simulink model "AnimationSpacecraftBodyVFC"  (R2020b)
settings: Solver=FixedStepDiscrete  StartTime=0.0  StopTime=inf  FixedStep=.1  RelTol=1e-3  EnableMultiTasking=on
InitFcn:
  | addpath('.')
libraries: simulink x6
settings Model: Creator=beard  LastModifiedBy=abdul
settings DataIOCC: LimitDataPoints=on  SaveFormat=Array  SignalLoggingSaveFormat=ModelDataLogs  ReturnWorkspaceOutputs=off
settings OptimizationCC: ExpressionDepthLimit=2147483647  InitFltsAndDblsToZero=on  LifeSpan=inf
settings DebuggingCC: UnderspecifiedInitializationDetection=Classic  MergeDetectMultiDrivingBlocksExec=none  SolverPrmCheckMsg=warning  FcnCallInpInsideContextMsg=warning  AllowSymbolicDim=off  StateNameClashWarn=warning  SFUnexpectedBacktrackingDiag=warning  SFNoUnconditionalDefaultTransitionDiag=warning  SFExecutionAtInitializationDiag=none  ArithmeticOperatorsInVariantConditions=warning
settings HardwareCC: ProdBitPerPointer=32  ProdBitPerSizeT=32  ProdBitPerPtrDiffT=32  ProdLargestAtomicFloat=None  ProdIntDivRoundTo=Undefined  ProdEndianess=Unspecified  ProdWordSize=32  ProdHWDeviceType=32-bit Generic
settings ModelReferenceCC: PropagateSignalLabelsOutOfModel=off
settings SFSimCC: SimUseLocalCustomCode=off  CustomCodeUndefinedFunction=UseInterfaceOnly
settings RTWCC: RTWUseLocalCustomCode=off
settings CodeAppCC: StateflowObjectComments=on
settings GRTTargetCC: TargetLangStandard=C89/C90 (ANSI)  CombineOutputUpdateFcns=off  GRTInterface=on
settings ConfigComp: CovMetricSettings=dw  CovSaveCumulativeToWorkspaceVar=on  CovSaveSingleToWorkspaceVar=on  CovExternalEMLEnable=off  CovSFcnEnable=off

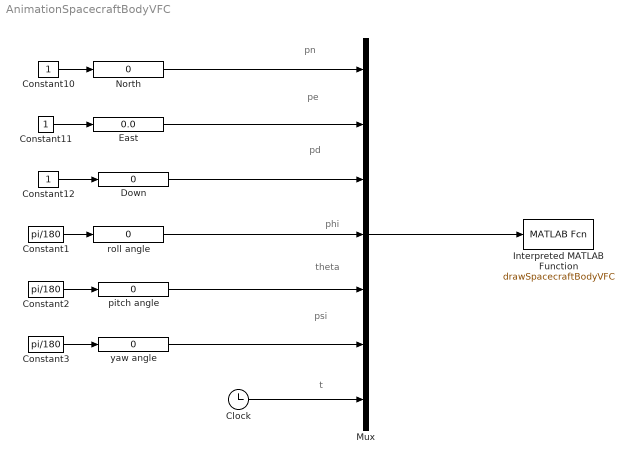
== system AnimationSpacecraftBodyVFC ==
  note: t
  note: pn
  note: pe
  note: pd
  note: phi
  note: theta
  note: psi
  Clock : Clock
  Constant1 : Constant  Value=pi/180
  Constant10 : Constant
  Constant11 : Constant
  Constant12 : Constant
  Constant2 : Constant  Value=pi/180
  Constant3 : Constant  Value=pi/180
  Down : simulink/Math Operations/Slider Gain  gain=0  low=-10  high=10
  East : simulink/Math Operations/Slider Gain  gain=0.0  low=-10  high=10
  Interpreted MATLAB Function : MATLABFcn  MATLABFcn=drawSpacecraftBodyVFC  OutputDimensions=0
  Mux : Mux  Inputs=7
  North : simulink/Math Operations/Slider Gain  gain=0  low=-10  high=10
  pitch angle : simulink/Math Operations/Slider Gain  gain=0  low=-180  high=180
  roll angle : simulink/Math Operations/Slider Gain  gain=0  low=-180  high=180
  "yaw angle " : simulink/Math Operations/Slider Gain  gain=0  low=-180  high=180
  wires:
  Mux/1 -> Interpreted MATLAB Function/1
  Constant1/1 -> roll angle/1
  Constant2/1 -> pitch angle/1
  Constant3/1 -> "yaw angle "/1
  Constant11/1 -> East/1
  Constant12/1 -> Down/1
  Constant10/1 -> North/1
  North/1 -> Mux/1
  East/1 -> Mux/2
  Down/1 -> Mux/3
  roll angle/1 -> Mux/4
  pitch angle/1 -> Mux/5
  "yaw angle "/1 -> Mux/6
  Clock/1 -> Mux/7
